simulink library "Launch_Vehicle_CL"  (R2019a)
settings: Solver=VariableStepAuto  StartTime=0.0  StopTime=10.0  RelTol=1e-3
undefined symbols (not defined in the file): ENV, Motor, VEH
libraries: Rail_UL x4
settings Model: Creator=jbore  LastModifiedBy=jbore

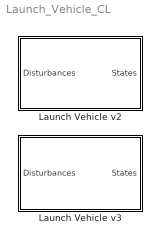
== system Launch_Vehicle_CL ==
  Launch Vehicle v2 : Subsystem
      mask Display:
      | patch([0 1 1 0], [0 0 1 1],[.8 1 1])
      | 
      | port_label('input',1,'\fontname{Cambria Math}Disturbances','texmode','on')
      | 
      | port_label('output',1,'\fontname{Cambria Math}States','texmode','on')
  Launch Vehicle v3 : Subsystem
      mask Display:
      | patch([0 1 1 0], [0 0 1 1],[.8 1 1])
      | 
      | port_label('input',1,'\fontname{Cambria Math}Disturbances','texmode','on')
      | 
      | port_label('output',1,'\fontname{Cambria Math}States','texmode','on')

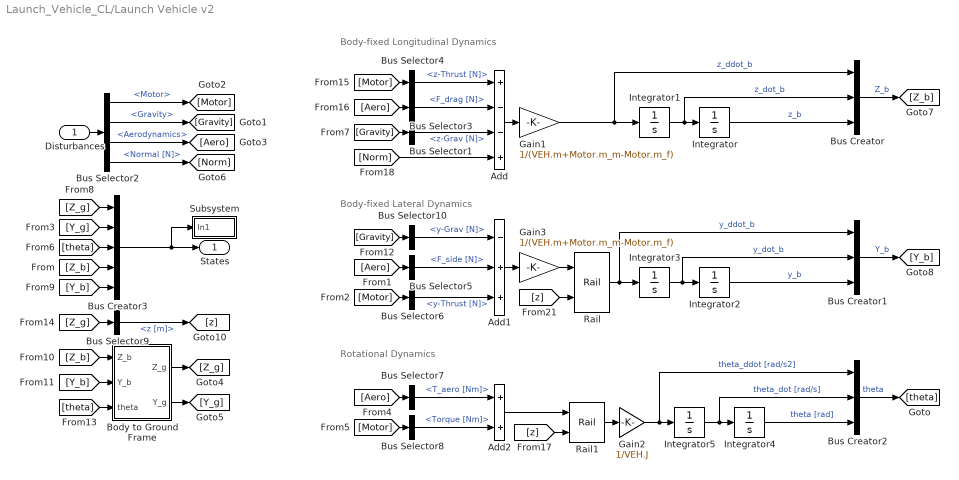
== system Launch_Vehicle_CL/Launch Vehicle v2 ==
  note: Rotational Dynamics
  note: Body-fixed Lateral Dynamics
  note: Body-fixed Longitudinal Dynamics
  Disturbances : Inport
  Add : Sum  Inputs=+--+
  Add1 : Sum  Inputs=-++
  Add2 : Sum
  Body to Ground Frame : Subsystem
      mask Display:
      | patch([0 1 1 0], [0 0 1 1],[.8 1 .8])
      | 
      | port_label('input',1,'\fontname{Cambria Math}b_z','texmode','on')
      | port_label('input',2,'\fontname{Cambria Math}b_y','texmode','on')
      | port_label('input',3,'\fontname{Cambria Math}\theta','texmode','on')
      | 
      | port_label('output',1,'\fontname{Cambria Math}g_z','texmode','on')
      | port_label('output',2,'\fontname{Cambria Math}g_y','texmode','on')
      | 
      | disp('\fontname{Cambria Math}\fontsize{12} R(\theta) ','texmode','on')
  Bus Creator : BusCreator  Inputs=3
  Bus Creator1 : BusCreator  Inputs=3
  Bus Creator2 : BusCreator  Inputs=3
  Bus Creator3 : BusCreator  Inputs=5
  Bus Selector1 : BusSelector  OutputSignals=z-Grav [N]
  Bus Selector10 : BusSelector  OutputSignals=y-Grav [N]
  Bus Selector2 : BusSelector  OutputSignals=Motor,Gravity,Aerodynamics,Normal [N]
  Bus Selector3 : BusSelector  OutputSignals=F_drag [N]
  Bus Selector4 : BusSelector  OutputSignals=z-Thrust [N]
  Bus Selector5 : BusSelector  OutputSignals=F_side [N]
  Bus Selector6 : BusSelector  OutputSignals=y-Thrust [N]
  Bus Selector7 : BusSelector  OutputSignals=T_aero [Nm]
  Bus Selector8 : BusSelector  OutputSignals=Torque [Nm]
  Bus Selector9 : BusSelector  OutputSignals=z [m]
  Gain1 : Gain  Gain=1/(VEH.m+Motor.m_m-Motor.m_f)
  Gain2 : Gain  Gain=1/VEH.J
  Gain3 : Gain  Gain=1/(VEH.m+Motor.m_m-Motor.m_f)
  Integrator : Integrator  LowerSaturationLimit=0
  Integrator{1..3,5} (4 alike) : Integrator
  Integrator4 : Integrator  InitialCondition=ENV.theta_0
  Rail : Rail_UL/Rail  z_r=ENV.z_r  t_b=Motor.t_b  a_out=0
  Rail1 : Rail_UL/Rail  z_r=ENV.z_r  t_b=Motor.t_b  a_out=0
  Subsystem : Subsystem
      mask Display:
      | patch([0 1 1 0], [0 0 1 1],[.8 1 .8])
      | 
      | 
      | 
      | disp('Log','texmode','on')
  States : Outport
  wires:
  [Norm] -> Add/4
  Bus Selector2/4 -> [Norm]  "<Normal [N]>"
  Gain2/1 -> Integrator5/1, Bus Creator2/1  "theta_ddot [rad/s2]"
  Disturbances/1 -> Bus Selector2/1
  Bus Creator/1 -> [Z_b]  "Z_b"
  Bus Creator1/1 -> [Y_b]  "Y_b"
  Bus Creator2/1 -> [theta]  "theta"
  Bus Creator3/1 -> Subsystem/1(In1), States/1
  [Z_g] -> Bus Creator3/1
  [Y_g] -> Bus Creator3/2
  [theta] -> Bus Creator3/3
  Bus Selector2/2 -> [Gravity]  "<Gravity>"
  Bus Selector2/1 -> [Motor]  "<Motor>"
  Bus Selector2/3 -> [Aero]  "<Aerodynamics>"
  Bus Selector3/1 -> Add/2  "<F_drag [N]>"
  Bus Selector4/1 -> Add/1  "<z-Thrust [N]>"
  Bus Selector5/1 -> Add1/2  "<F_side [N]>"
  Bus Selector6/1 -> Add1/3  "<y-Thrust [N]>"
  [Motor] -> Bus Selector8/1
  [Aero] -> Bus Selector7/1
  Bus Selector8/1 -> Add2/2  "<Torque [Nm]>"
  Bus Selector7/1 -> Add2/1  "<T_aero [Nm]>"
  Add/1 -> Gain1/1
  Add1/1 -> Gain3/1
  [z] -> Rail/2
  Integrator5/1 -> Bus Creator2/2, Integrator4/1  "theta_dot [rad/s]"
  Integrator4/1 -> Bus Creator2/3  "theta [rad]"
  Rail1/1 -> Gain2/1
  [z] -> Rail1/2
  Add2/1 -> Rail1/1
  Gain3/1 -> Rail/1
  Rail/1 -> Bus Creator1/1, Integrator3/1  "y_ddot_b"
  Gain1/1 -> Bus Creator/1, Integrator1/1  "z_ddot_b"
  Integrator1/1 -> Bus Creator/2, Integrator/1  "z_dot_b"
  Integrator3/1 -> Bus Creator1/2, Integrator2/1  "y_dot_b"
  Integrator2/1 -> Bus Creator1/3  "y_b"
  Integrator/1 -> Bus Creator/3  "z_b"
  [Y_b] -> Bus Creator3/5
  [Z_b] -> Bus Creator3/4
  [Z_b] -> Body to Ground Frame/1(Z_b)
  [Y_b] -> Body to Ground Frame/2(Y_b)
  [theta] -> Body to Ground Frame/3(theta)
  Body to Ground Frame/2(Y_g) -> [Y_g]
  Body to Ground Frame/1(Z_g) -> [Z_g]
  [Z_g] -> Bus Selector9/1
  Bus Selector9/1 -> [z]  "<z [m]>"
  Bus Selector1/1 -> Add/3  "<z-Grav [N]>"
  Bus Selector10/1 -> Add1/1  "<y-Grav [N]>"
  [Gravity] -> Bus Selector1/1
  [Motor] -> Bus Selector4/1
  [Gravity] -> Bus Selector10/1
  [Aero] -> Bus Selector3/1
  [Motor] -> Bus Selector6/1
  [Aero] -> Bus Selector5/1

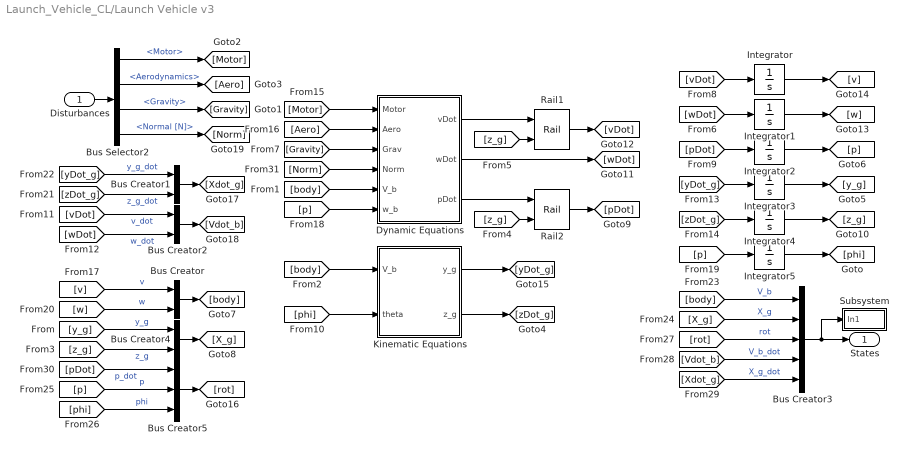
== system Launch_Vehicle_CL/Launch Vehicle v3 ==
  Disturbances : Inport
  Bus Creator{,1..2,4} (4 alike) : BusCreator  Inputs=2
  Bus Creator3 : BusCreator  Inputs=5
  Bus Creator5 : BusCreator  Inputs=3
  Bus Selector2 : BusSelector  OutputSignals=Motor,Aerodynamics,Gravity,Normal [N]
  Dynamic Equations : MATLAB Function  TreatAsAtomicUnit=on
  Integrator{,1..3} (4 alike) : Integrator
  Integrator4 : Integrator  LimitOutput=on  LowerSaturationLimit=0
  Integrator5 : Integrator  InitialCondition=ENV.phi_0
  Kinematic Equations : MATLAB Function  TreatAsAtomicUnit=on
  Rail1 : Rail_UL/Rail  z_r=ENV.z_r  t_b=Motor.t_b  a_out=0
  Rail2 : Rail_UL/Rail  z_r=ENV.z_r  t_b=Motor.t_b  a_out=0
  Subsystem : Subsystem
      mask Display:
      | patch([0 1 1 0], [0 0 1 1],[.8 1 .8])
      | 
      | 
      | 
      | disp('Log','texmode','on')
  States : Outport
  wires:
  [Norm] -> Dynamic Equations/4(Norm)
  Bus Selector2/4 -> [Norm]  "<Normal [N]>"
  [zDot_g] -> Bus Creator1/2  "z_g_dot"
  Bus Creator4/1 -> [X_g]
  [yDot_g] -> Bus Creator1/1  "y_g_dot"
  [vDot] -> Integrator/1
  [p] -> Dynamic Equations/6(w_b)
  [Vdot_b] -> Bus Creator3/4  "V_b_dot"
  Bus Creator2/1 -> [Vdot_b]
  Rail1/1 -> [vDot]
  [vDot] -> Bus Creator2/1  "v_dot"
  [z_g] -> Rail1/2
  Bus Creator5/1 -> [rot]
  [z_g] -> Rail2/2
  [z_g] -> Bus Creator4/2  "z_g"
  Bus Creator/1 -> [body]
  Bus Selector2/1 -> [Motor]  "<Motor>"
  Kinematic Equations/1(y_g) -> [yDot_g]
  [y_g] -> Bus Creator4/1  "y_g"
  [wDot] -> Bus Creator2/2  "w_dot"
  [Motor] -> Dynamic Equations/1(Motor)
  [p] -> Integrator5/1
  Dynamic Equations/1(vDot) -> Rail1/1
  [rot] -> Bus Creator3/3  "rot"
  Integrator3/1 -> [y_g]
  [w] -> Bus Creator/2  "w"
  Kinematic Equations/2(z_g) -> [zDot_g]
  Bus Creator1/1 -> [Xdot_g]
  Integrator4/1 -> [z_g]
  [p] -> Bus Creator5/2  "p"
  [phi] -> Kinematic Equations/2(theta)
  [body] -> Bus Creator3/1  "V_b"
  [v] -> Bus Creator/1  "v"
  [yDot_g] -> Integrator3/1
  [pDot] -> Integrator2/1
  Integrator/1 -> [v]
  [zDot_g] -> Integrator4/1
  Dynamic Equations/2(wDot) -> [wDot]
  [Gravity] -> Dynamic Equations/3(Grav)
  [phi] -> Bus Creator5/3  "phi"
  Integrator5/1 -> [phi]
  [pDot] -> Bus Creator5/1  "p_dot"
  Integrator1/1 -> [w]
  Rail2/1 -> [pDot]
  Bus Selector2/3 -> [Gravity]  "<Gravity>"
  [body] -> Kinematic Equations/1(V_b)
  [X_g] -> Bus Creator3/2  "X_g"
  [body] -> Dynamic Equations/5(V_b)
  [Aero] -> Dynamic Equations/2(Aero)
  Bus Creator3/1 -> Subsystem/1(In1), States/1
  Integrator2/1 -> [p]
  [Xdot_g] -> Bus Creator3/5  "X_g_dot"
  Dynamic Equations/3(pDot) -> Rail2/1
  Disturbances/1 -> Bus Selector2/1
  Bus Selector2/2 -> [Aero]  "<Aerodynamics>"
  [wDot] -> Integrator1/1

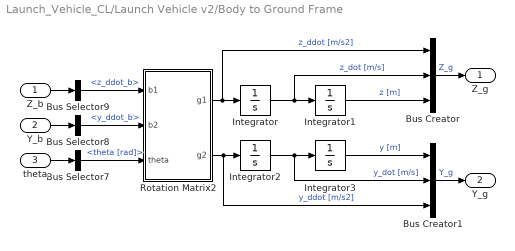
== system Launch_Vehicle_CL/Launch Vehicle v2/Body to Ground Frame ==
  Z_b : Inport
  Y_b : Inport  Port=2
  theta : Inport  Port=3
  Bus Creator : BusCreator  Inputs=3
  Bus Creator1 : BusCreator  Inputs=3
  Bus Selector7 : BusSelector  OutputSignals=theta [rad]
  Bus Selector8 : BusSelector  OutputSignals=y_ddot_b
  Bus Selector9 : BusSelector  OutputSignals=z_ddot_b
  Integrator : Integrator
  Integrator1 : Integrator  LimitOutput=on  LowerSaturationLimit=0
  Integrator2 : Integrator
  Integrator3 : Integrator
  Rotation Matrix2 : MATLAB Function  TreatAsAtomicUnit=on
  Z_g : Outport
  Y_g : Outport  Port=2
  wires:
  Y_b/1 -> Bus Selector8/1
  Bus Selector7/1 -> Rotation Matrix2/3(theta)  "<theta [rad]>"
  Z_b/1 -> Bus Selector9/1
  theta/1 -> Bus Selector7/1
  Bus Selector8/1 -> Rotation Matrix2/2(b2)  "<y_ddot_b>"
  Bus Selector9/1 -> Rotation Matrix2/1(b1)  "<z_ddot_b>"
  Bus Creator1/1 -> Y_g/1  "Y_g"
  Bus Creator/1 -> Z_g/1  "Z_g"
  Rotation Matrix2/1(g1) -> Bus Creator/1, Integrator/1  "z_ddot [m/s2]"
  Integrator3/1 -> Bus Creator1/1  "y [m]"
  Rotation Matrix2/2(g2) -> Bus Creator1/3, Integrator2/1  "y_ddot [m/s2]"
  Integrator2/1 -> Bus Creator1/2, Integrator3/1  "y_dot [m/s]"
  Integrator/1 -> Bus Creator/2, Integrator1/1  "z_dot [m/s]"
  Integrator1/1 -> Bus Creator/3  "z [m]"

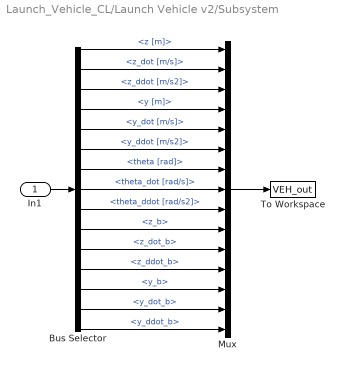
== system Launch_Vehicle_CL/Launch Vehicle v2/Subsystem ==
  In1 : Inport
  Bus Selector : BusSelector  OutputSignals=Z_g.z [m],Z_g.z_dot [m/s],Z_g.z_ddot [m/s2],Y_g.y [m],Y_g.y_dot [m/s],Y_g.y_ddot [m/s2],theta.theta [rad],theta.theta_dot [rad/s],theta.theta_ddot [rad/s2],Z_b.z_b,Z_b.z_dot_b,Z_b.z_ddot_b,Y_b.y_b,Y_b.y_dot_b,Y_b.y_ddot_b
  Mux : Mux  Inputs=15
  To Workspace : ToWorkspace  VariableName=VEH_out  SaveFormat=Structure With Time  SampleTime=-1
  wires:
  In1/1 -> Bus Selector/1
  Mux/1 -> To Workspace/1
  Bus Selector/1 -> Mux/1  "<z [m]>"
  Bus Selector/2 -> Mux/2  "<z_dot [m/s]>"
  Bus Selector/3 -> Mux/3  "<z_ddot [m/s2]>"
  Bus Selector/4 -> Mux/4  "<y [m]>"
  Bus Selector/5 -> Mux/5  "<y_dot [m/s]>"
  Bus Selector/6 -> Mux/6  "<y_ddot [m/s2]>"
  Bus Selector/7 -> Mux/7  "<theta [rad]>"
  Bus Selector/8 -> Mux/8  "<theta_dot [rad/s]>"
  Bus Selector/9 -> Mux/9  "<theta_ddot [rad/s2]>"
  Bus Selector/10 -> Mux/10  "<z_b>"
  Bus Selector/11 -> Mux/11  "<z_dot_b>"
  Bus Selector/12 -> Mux/12  "<z_ddot_b>"
  Bus Selector/13 -> Mux/13  "<y_b>"
  Bus Selector/14 -> Mux/14  "<y_dot_b>"
  Bus Selector/15 -> Mux/15  "<y_ddot_b>"

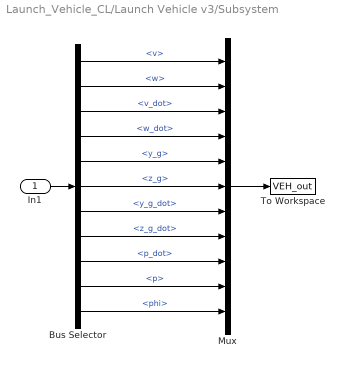
== system Launch_Vehicle_CL/Launch Vehicle v3/Subsystem ==
  In1 : Inport
  Bus Selector : BusSelector  OutputSignals=V_b.v,V_b.w,V_b_dot.v_dot,V_b_dot.w_dot,X_g.y_g,X_g.z_g,X_g_dot.y_g_dot,X_g_dot.z_g_dot,rot.p_dot,rot.p,rot.phi
  Mux : Mux  Inputs=11
  To Workspace : ToWorkspace  VariableName=VEH_out  SaveFormat=Structure With Time  SampleTime=-1
  wires:
  Bus Selector/11 -> Mux/11  "<phi>"
  Bus Selector/10 -> Mux/10  "<p>"
  Bus Selector/9 -> Mux/9  "<p_dot>"
  Bus Selector/8 -> Mux/8  "<z_g_dot>"
  Bus Selector/7 -> Mux/7  "<y_g_dot>"
  Bus Selector/6 -> Mux/6  "<z_g>"
  Bus Selector/5 -> Mux/5  "<y_g>"
  Bus Selector/4 -> Mux/4  "<w_dot>"
  Bus Selector/3 -> Mux/3  "<v_dot>"
  Bus Selector/2 -> Mux/2  "<w>"
  Bus Selector/1 -> Mux/1  "<v>"
  Mux/1 -> To Workspace/1
  In1/1 -> Bus Selector/1

== matlab function Launch_Vehicle_CL/Launch Vehicle v3/Dynamic Equations ==
  data: Motor input size=5; vDot output; wDot output; Aero input size=6; Grav input size=5; Norm input; V_b input; w_b input; pDot output
function [vDot,wDot,pDot] = fcn(Motor,Aero,Grav,Norm,V_b,w_b)

F_t = [Motor(3) Motor(2)]';
F_a = [Aero(2) Aero(1)]';
F_g = [Grav(3) Grav(1)]';
T_t = Motor(4);
T_a = Aero(3);

m = Grav(4);
J = Grav(5);

v = V_b(1);
w = V_b(2);

vDot = -w*w_b+1/m*(F_t(1)+F_g(1)+F_a(1));
wDot = v*w_b+1/m*(F_t(2)-F_g(2)-F_a(2)+Norm);
pDot = 1/J*(T_t+T_a);

== matlab function Launch_Vehicle_CL/Launch Vehicle v2/Body to Ground Frame/Rotation Matrix2 ==
  data: b1 input; b2 input; g1 output; theta input; g2 output
function [g1,g2]= fcn(b1,b2,theta)
%#codegen

B = [b1;b2];
R = [cos(theta) sin(theta);-sin(theta) cos(theta)];
G = R*B;
g1 = G(1);
g2 = G(2);

== matlab function Launch_Vehicle_CL/Launch Vehicle v3/Kinematic Equations ==
  data: V_b input size=2; theta input; y_g output; z_g output
function [y_g,z_g] = fcn(V_b,theta)

V_b = [V_b(1) V_b(2)]';
R = [cos(theta) -sin(theta);sin(theta) cos(theta)];
V_g = R*V_b;
y_g = V_g(1);
z_g = V_g(2);
